simulink library "thrAttachPtKinematics_ul"  (R2018b)
settings: Solver=VariableStepAuto  StartTime=0.0  StopTime=10.0  RelTol=1e-3
undefined symbols (not defined in the file or in its folder): gndStnMmtArms
libraries: firstOrdTrnsThm_ul x1
settings Model: Creator=mcobb  LastModifiedBy=mcobb

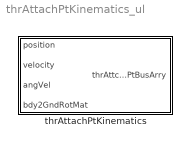
== system thrAttachPtKinematics_ul ==
  thrAttachPtKinematics : Subsystem  mask{atchPts=gndStnMmtArms}
      mask prompts: atchPts "Thether attachment point vec in platform frame"
      mask init:
      | thrAttachPtKinematics_init

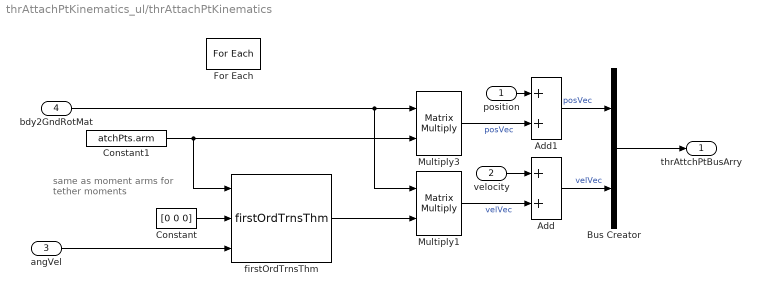
== system thrAttachPtKinematics_ul/thrAttachPtKinematics ==
  note: same as moment arms
      | for tether moments
  position : Inport
  velocity : Inport  Port=2
  angVel : Inport  Port=3
  bdy2GndRotMat : Inport  Port=4
  Add : Sum
  Add1 : Sum
  Bus Creator : BusCreator  Inputs=2  OutDataTypeStr=Bus: thrAttachPtKinematicsBus  NonVirtualBus=on
  Constant : Constant  Value=[0 0 0]
  Constant1 : Constant  Value=atchPts.arm
  For Each : ForEach  DisableCoverage=on  IterateSubsysMaskParameter=on  SubsysMaskParameterIterationDimension=2  IndexMode=One-based
  Multiply1 : Product  Multiplication=Matrix(*)
  Multiply3 : Product  Multiplication=Matrix(*)
  firstOrdTrnsThm : firstOrdTrnsThm_ul/firstOrdTrnsThm  SystemSampleTime=-1
  thrAttchPtBusArry : Outport  ConcatenationDimension=1
  wires:
  Add1/1 -> Bus Creator/1  "posVec"
  Add/1 -> Bus Creator/2  "velVec"
  bdy2GndRotMat/1 -> Multiply3/1, Multiply1/1
  Constant/1 -> firstOrdTrnsThm/2
  firstOrdTrnsThm/1 -> Multiply1/2
  angVel/1 -> firstOrdTrnsThm/3
  Constant1/1 -> Multiply3/2, firstOrdTrnsThm/1
  Bus Creator/1 -> thrAttchPtBusArry/1
  position/1 -> Add1/1
  velocity/1 -> Add/1
  Multiply1/1 -> Add/2  "velVec"
  Multiply3/1 -> Add1/2  "posVec"
